simulink model "test8"  (R2014b)
settings: Solver=ode45  StartTime=0.0  StopTime=.4  RelTol=1e-3
libraries: dspswit3 x4, siglabs_lib x1, commrandsrc2 x1
settings Model: Creator=Ben  LastModifiedBy=Ben

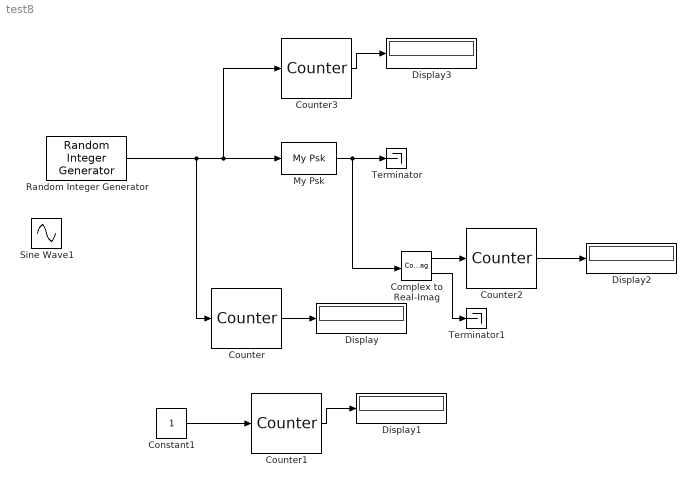
== system test8 ==
  Complex to Real-Imag : ComplexToRealImag
  Constant1 : Constant  SampleTime=.1
  Counter{,1..3} (4 alike) : dspswit3/Counter  Direction=Up  CountEvent=Non-zero sample  CounterSize=User defined  MaxCount=999999999999  InitialCount=0  Output=Count  HitValue=32  ResetInput=off  SamplesPerFrame=1  Ts=1  CntDtype=double  HitDtype=Logical
  Display{,1..3} (4 alike) : Display
  My Psk : siglabs_lib/My Psk  SampsPerSym=2
  Random Integer Generator : commrandsrc2/Random Integer Generator  mul=4  seed=37  Ts=.1  frameBased=off  sampPerFrame=1  orient=off  outDataType=double
  Sine Wave1 : Sin  Frequency=2.1  SampleTime=.1
  Terminator : Terminator
  Terminator1 : Terminator
  wires:
  Random Integer Generator/1 -> Counter/1, My Psk/1, Counter3/1
  My Psk/1 -> Complex to Real-Imag/1, Terminator/1
  Counter/1 -> Display/1
  Constant1/1 -> Counter1/1
  Counter1/1 -> Display1/1
  Counter2/1 -> Display2/1
  Complex to Real-Imag/1 -> Counter2/1
  Complex to Real-Imag/2 -> Terminator1/1
  Counter3/1 -> Display3/1
